simulink model "Robot_PID_model"  (R2016b)
settings: Solver=VariableStepAuto  StartTime=0.0  StopTime=10.0  RelTol=1e-3
values from neighbouring files (symbols this model uses):
  A = [0, 0, 1, 0 ... (first row only)    [Robot_PID.m]    (also in Robot_PID2.m)
  B = [0 ... (first row only)    [Robot_PID.m]    (also in Robot_PID2.m)
  C = [1,0,0,0 ... (first row only)    [Robot_PID.m]    (also in Robot_PID2.m)
  D = [0,0,0,0]'    [Robot_PID.m]    (also in Robot_PID2.m)
  Kd = 0.1    [Robot_PID.m]
  Ki = 100    [Robot_PID.m]
  Kp = 10    [Robot_PID.m]
  Phi_0 = 0    [Robot_PID.m]
  Phi_y = 0    [Robot_PID.m]
  R = 0.04    [Robot_PID.m]    (also in Robot_PID2.m)
libraries: simulink x1
settings Model: Creator=macbookmichal  LastModifiedBy=macbookmichal

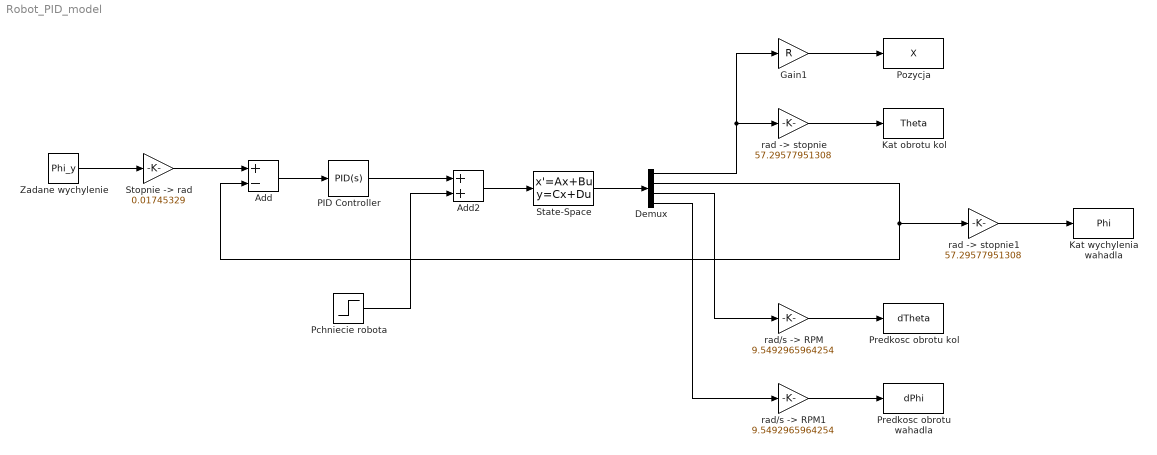
== system Robot_PID_model ==
  Add : Sum  Inputs=+-
  Add2 : Sum
  Demux : Demux
  Gain1 : Gain  Gain=R
  Kat obrotu kol : ToWorkspace  VariableName=Theta  SampleTime=-1
  Kat wychylenia wahadla : ToWorkspace  VariableName=Phi  SampleTime=-1
  PID Controller : simulink/Continuous/PID Controller  Controller=PID  TimeDomain=Continuous-time  SampleTime=-1  IntegratorMethod=Forward Euler  FilterMethod=Forward Euler  Form=Parallel  UseFilter=on  ControllerParametersSource=internal  P=Kp  I=Ki  D=Kd  N=100  InitialConditionSource=internal  InitialConditionForIntegrator=0  InitialConditionForFilter=0  ExternalReset=none  LimitOutput=off  UpperSaturationLimit=inf  LowerSaturationLimit=-inf  LinearizeAsGain=on  AntiWindupMode=none  Kb=1  TrackingMode=off  Kt=1  PParamMin=[]  PParamMax=[]  IParamMin=[]  IParamMax=[]  DParamMin=[]  DParamMax=[]  NParamMin=[]  NParamMax=[]  KbParamMin=[]  KbParamMax=[]  KtParamMin=[]  KtParamMax=[]  POutMin=[]  POutMax=[]  IOutMin=[]  IOutMax=[]  DOutMin=[]  DOutMax=[]  NOutMin=[]  NOutMax=[]  KbOutMin=[]  KbOutMax=[]  KtOutMin=[]  KtOutMax=[]  IntegratorOutMin=[]  IntegratorOutMax=[]  FilterOutMin=[]  FilterOutMax=[]  SumOutMin=[]  SumOutMax=[]  SumI1OutMin=[]  SumI1OutMax=[]  SumI2OutMin=[]  SumI2OutMax=[]  SumI3OutMin=[]  SumI3OutMax=[]  SumDOutMin=[]  SumDOutMax=[]  SaturationOutMin=[]  SaturationOutMax=[]  IntegratorContinuousStateAttributes=''  IntegratorStateMustResolveToSignalObject=off  IntegratorRTWStateStorageClass=Auto  FilterContinuousStateAttributes=''  FilterStateMustResolveToSignalObject=off  FilterRTWStateStorageClass=Auto  DifferentiatorICPrevScaledInput=0  DifferentiatorOutMin=[]  DifferentiatorOutMax=[]
  Pchniecie robota : Step  After=0.25  SampleTime=0
  Pozycja : ToWorkspace  VariableName=X  SampleTime=-1
  Predkosc obrotu kol : ToWorkspace  VariableName=dTheta  SampleTime=-1
  Predkosc obrotu wahadla : ToWorkspace  VariableName=dPhi  SampleTime=-1
  State-Space : StateSpace  A=A  B=B  C=C  D=D  X0=Phi_0 * 0.01745329
  "Stopnie -> rad" : Gain  Gain=0.01745329
  Zadane wychylenie : Constant  Value=Phi_y
  "rad -> stopnie" : Gain  Gain=57.29577951308
  "rad -> stopnie1" : Gain  Gain=57.29577951308
  "rad/s -> RPM" : Gain  Gain=9.5492965964254
  "rad/s -> RPM1" : Gain  Gain=9.5492965964254
  wires:
  Zadane wychylenie/1 -> "Stopnie -> rad"/1
  Add/1 -> PID Controller/1
  State-Space/1 -> Demux/1
  Demux/1 -> "rad -> stopnie"/1, Gain1/1
  Gain1/1 -> Pozycja/1
  Demux/3 -> "rad/s -> RPM"/1
  Demux/4 -> "rad/s -> RPM1"/1
  "Stopnie -> rad"/1 -> Add/1
  "rad -> stopnie"/1 -> Kat obrotu kol/1
  "rad -> stopnie1"/1 -> Kat wychylenia wahadla/1
  "rad/s -> RPM"/1 -> Predkosc obrotu kol/1
  "rad/s -> RPM1"/1 -> Predkosc obrotu wahadla/1
  Pchniecie robota/1 -> Add2/2
  Add2/1 -> State-Space/1
  PID Controller/1 -> Add2/1
  Demux/2 -> Add/2, "rad -> stopnie1"/1
